simulink model "psc"  (R2023b)
settings: Solver=VariableStepAuto  StartTime=0.0  StopTime=.1  RelTol=1e-3
undefined symbols (not defined in the file): DiscIntNeverNeededParam, f_sw, K_p, L_f, L_g, R_a, R_L, T_s, U_dc, u_gN, w_b, w_g
libraries: simulink x1
settings Model: Creator=maatt  LastModifiedBy=maatt
settings DataIOCC: ReturnWorkspaceOutputs=off

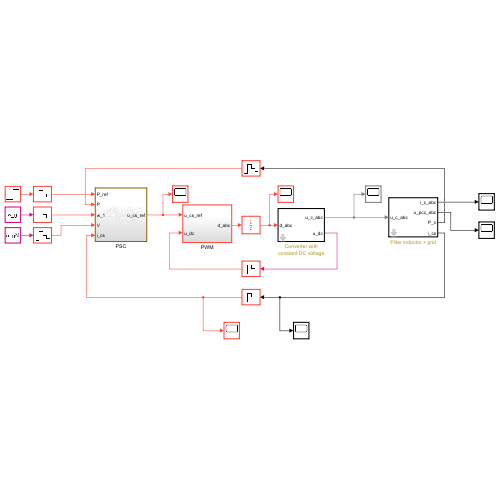
[thumbnail: Simulink's stored preview of the top-level diagram]
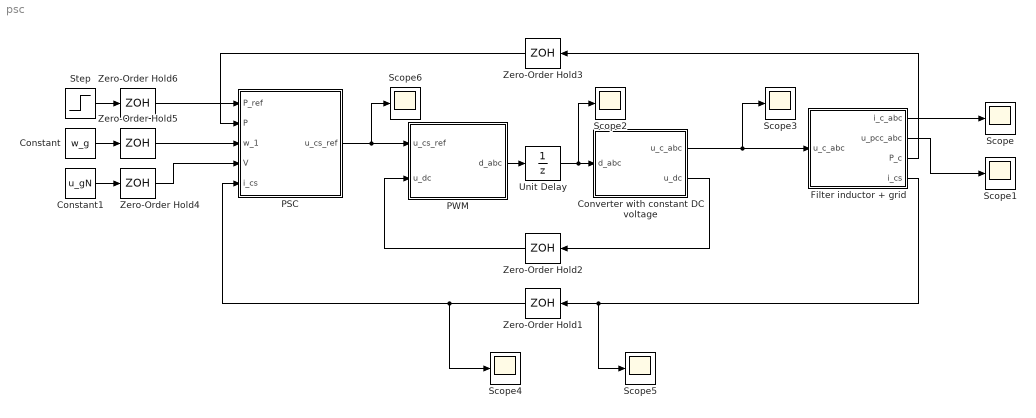
== system psc ==
  Constant : Constant  Value=w_g
  Constant1 : Constant  Value=u_gN
  "Converter with constant DC voltage " : Subsystem  mask{f_sw=f_sw, u_dc=U_dc}
      mask prompts: f_sw "Switching frequency (Hz)"; u_dc "DC-bus voltage (V)"
      mask init:
      | T_s = 1/(2*f_sw);
  Filter inductor + grid : Subsystem  mask{L_f=L_f, L_g=L_g, R_L=R_L}
      mask prompts: L_f "Filter inductance (H)"; L_g "Grid inductance (H)"; R_L "Series resistance (ohm)"
  PSC : Subsystem
  PWM : Subsystem
  Scope{,1..6} (7 alike) : Scope
  Step : Step  Time=.04  After=20  SampleTime=T_s
  Unit Delay : UnitDelay  SampleTime=T_s  HasFrameUpgradeWarning=on
  Zero-Order Hold{1..6} (6 alike) : ZeroOrderHold  SampleTime=T_s
  wires:
  "Converter with constant DC voltage "/1(u_c_abc) -> Scope3/1, Filter inductor + grid/1(u_c_abc)
  PWM/1(d_abc) -> Unit Delay/1
  PSC/1(u_cs_ref) -> Scope6/1, PWM/1(u_cs_ref)
  "Converter with constant DC voltage "/2(u_dc) -> Zero-Order Hold2/1
  Step/1 -> Zero-Order Hold6/1
  Constant/1 -> Zero-Order Hold5/1
  Constant1/1 -> Zero-Order Hold4/1
  Filter inductor + grid/1(i_c_abc) -> Scope/1
  Filter inductor + grid/2(u_pcc_abc) -> Scope1/1
  Filter inductor + grid/3(P_c) -> Zero-Order Hold3/1
  Filter inductor + grid/4(i_cs) -> Scope5/1, Zero-Order Hold1/1
  Unit Delay/1 -> Scope2/1, "Converter with constant DC voltage "/1(d_abc)
  Zero-Order Hold1/1 -> Scope4/1, PSC/5(i_cs)
  Zero-Order Hold2/1 -> PWM/2(u_dc)
  Zero-Order Hold3/1 -> PSC/2(P)
  Zero-Order Hold4/1 -> PSC/4(V)
  Zero-Order Hold5/1 -> PSC/3(w_1)
  Zero-Order Hold6/1 -> PSC/1(P_ref)

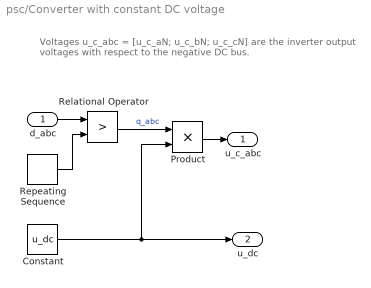
== system psc/Converter with constant DC voltage  ==
  note: Voltages u_c_abc = [u_c_aN; u_c_bN; u_c_cN] are the inverter
      | output voltages with respect to the negative DC bus.
  d_abc : Inport
  Constant : Constant  Value=u_dc
  Product : Product
  Relational Operator : RelationalOperator  Operator=>  OutDataTypeStr='double'  InputSameDT=off
  Repeating Sequence : simulink/Sources/Repeating Sequence  rep_seq_t=[0 1 2]*T_s  rep_seq_y=[1 0 1]
  u_c_abc : Outport
  u_dc : Outport  Port=2
  wires:
  Repeating Sequence/1 -> Relational Operator/2
  d_abc/1 -> Relational Operator/1
  Product/1 -> u_c_abc/1
  Relational Operator/1 -> Product/1  "q_abc"
  Constant/1 -> Product/2, u_dc/1

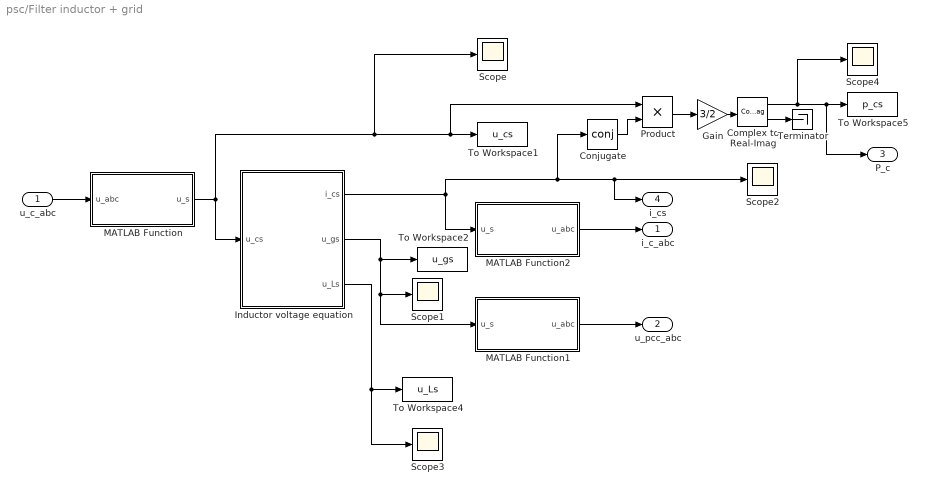
== system psc/Filter inductor + grid ==
  u_c_abc : Inport
  Complex to Real-Imag : ComplexToRealImag
  Conjugate : Math  Operator=conj  SignedPower=on  RndMeth=Zero
  Gain : Gain  Gain=3/2
  Inductor voltage equation : Subsystem
  MATLAB Function : MATLAB Function  TreatAsAtomicUnit=on
  MATLAB Function1 : MATLAB Function  TreatAsAtomicUnit=on
  MATLAB Function2 : MATLAB Function  TreatAsAtomicUnit=on
  Product : Product
  Scope{,1..4} (5 alike) : Scope
  Terminator : Terminator
  To Workspace1 : ToWorkspace  VariableName=u_cs  SaveFormat=Timeseries
  To Workspace2 : ToWorkspace  VariableName=u_gs  SaveFormat=Timeseries
  To Workspace4 : ToWorkspace  VariableName=u_Ls  SaveFormat=Timeseries
  To Workspace5 : ToWorkspace  VariableName=p_cs  SaveFormat=Timeseries
  i_c_abc : Outport
  u_pcc_abc : Outport  Port=2
  P_c : Outport  Port=3
  i_cs : Outport  Port=4
  wires:
  u_c_abc/1 -> MATLAB Function/1(u_abc)
  Inductor voltage equation/1(i_cs) -> i_cs/1, Scope2/1, Conjugate/1, MATLAB Function2/1(u_s)
  MATLAB Function2/1(u_abc) -> i_c_abc/1
  MATLAB Function/1(u_s) -> Inductor voltage equation/1(u_cs), Scope/1, Product/1, To Workspace1/1
  Inductor voltage equation/2(u_gs) -> Scope1/1, MATLAB Function1/1(u_s), To Workspace2/1
  Inductor voltage equation/3(u_Ls) -> To Workspace4/1, Scope3/1
  MATLAB Function1/1(u_abc) -> u_pcc_abc/1
  Conjugate/1 -> Product/2
  Complex to Real-Imag/1 -> Scope4/1, P_c/1, To Workspace5/1
  Complex to Real-Imag/2 -> Terminator/1
  Product/1 -> Gain/1
  Gain/1 -> Complex to Real-Imag/1

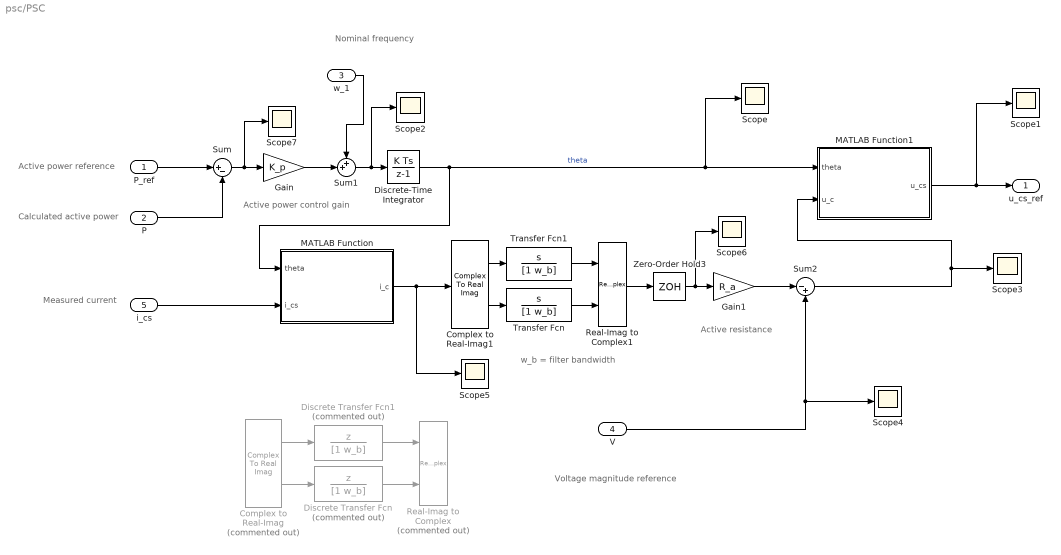
== system psc/PSC ==
  note: Active resistance
  note: Active power reference
  note: Calculated active power
  note: Measured current
  note: Nominal frequency
  note: Voltage magnitude reference
  note: Active power control gain
  note: w_b = filter bandwidth
  P_ref : Inport
  P : Inport  Port=2
  w_1 : Inport  Port=3
  V : Inport  Port=4
  i_cs : Inport  Port=5
  Complex to Real-Imag : ComplexToRealImag  Commented=on
  Complex to Real-Imag1 : ComplexToRealImag
  Discrete Transfer Fcn : DiscreteTransferFcn  Commented=on  Numerator=[1 0]  Denominator=[1 w_b]
  Discrete Transfer Fcn1 : DiscreteTransferFcn  Commented=on  Numerator=[1 0]  Denominator=[1 w_b]
  Discrete-Time Integrator : DiscreteIntegrator  SampleTime=T_s  OutMin=[-pi]  OutMax=[pi]  ICPrevOutput=DiscIntNeverNeededParam  ICPrevScaledInput=DiscIntNeverNeededParam
  Gain : Gain  Gain=K_p
  Gain1 : Gain  Gain=R_a
  MATLAB Function : MATLAB Function  TreatAsAtomicUnit=on
  MATLAB Function1 : MATLAB Function  TreatAsAtomicUnit=on
  Real-Imag to Complex : RealImagToComplex  Commented=on
  Real-Imag to Complex1 : RealImagToComplex
  Scope{,1..7} (8 alike) : Scope
  Sum : Sum  Inputs=|+-
  Sum1 : Sum  Inputs=++|
  Sum2 : Sum  Inputs=|-+
  Transfer Fcn : TransferFcn  Numerator=[1 0]  Denominator=[1 w_b]
  Transfer Fcn1 : TransferFcn  Numerator=[1 0]  Denominator=[1 w_b]
  Zero-Order Hold3 : ZeroOrderHold  SampleTime=T_s
  u_cs_ref : Outport
  wires:
  P_ref/1 -> Sum/1
  P/1 -> Sum/2
  Sum/1 -> Scope7/1, Gain/1
  Gain/1 -> Sum1/2
  w_1/1 -> Sum1/1
  Sum1/1 -> Discrete-Time Integrator/1, Scope2/1
  Discrete-Time Integrator/1 -> Scope/1, MATLAB Function1/1(theta), MATLAB Function/1(theta)  "theta"
  Gain1/1 -> Sum2/1
  V/1 -> Scope4/1, Sum2/2
  Sum2/1 -> MATLAB Function1/2(u_c), Scope3/1
  MATLAB Function1/1(u_cs) -> Scope1/1, u_cs_ref/1
  i_cs/1 -> MATLAB Function/2(i_cs)
  Complex to Real-Imag/1 -> Discrete Transfer Fcn1/1
  Complex to Real-Imag/2 -> Discrete Transfer Fcn/1
  MATLAB Function/1(i_c) -> Complex to Real-Imag1/1, Scope5/1
  Discrete Transfer Fcn/1 -> Real-Imag to Complex/2
  Discrete Transfer Fcn1/1 -> Real-Imag to Complex/1
  Transfer Fcn1/1 -> Real-Imag to Complex1/1
  Transfer Fcn/1 -> Real-Imag to Complex1/2
  Complex to Real-Imag1/2 -> Transfer Fcn/1
  Complex to Real-Imag1/1 -> Transfer Fcn1/1
  Zero-Order Hold3/1 -> Scope6/1, Gain1/1
  Real-Imag to Complex1/1 -> Zero-Order Hold3/1

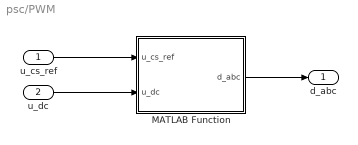
== system psc/PWM ==
  u_cs_ref : Inport
  u_dc : Inport  Port=2
  MATLAB Function : MATLAB Function  TreatAsAtomicUnit=on
  d_abc : Outport
  wires:
  u_cs_ref/1 -> MATLAB Function/1(u_cs_ref)
  MATLAB Function/1(d_abc) -> d_abc/1
  u_dc/1 -> MATLAB Function/2(u_dc)

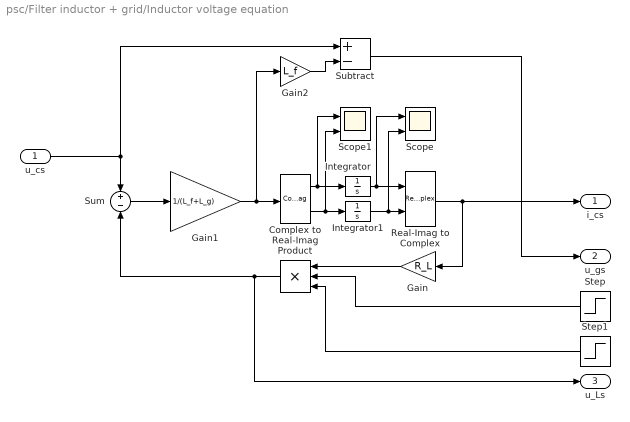
== system psc/Filter inductor + grid/Inductor voltage equation ==
  u_cs : Inport
  Complex to Real-Imag : ComplexToRealImag
  Gain : Gain  Gain=R_L
  Gain1 : Gain  Gain=1/(L_f+L_g)
  Gain2 : Gain  Gain=L_f
  Integrator : Integrator
  Integrator1 : Integrator
  Product : Product  Inputs=3
  Real-Imag to Complex : RealImagToComplex
  Scope : Scope  NumInputPorts=2
  Scope1 : Scope  NumInputPorts=2
  Step : Step  Time=0.05  Before=1  After=2  SampleTime=0
  Step1 : Step  Time=0.08  Before=1  SampleTime=0
  Subtract : Sum  Inputs=+-
  Sum : Sum  Inputs=+|-
  i_cs : Outport
  u_gs : Outport  Port=2
  u_Ls : Outport  Port=3
  wires:
  u_cs/1 -> Subtract/1, Sum/1
  Sum/1 -> Gain1/1
  Gain1/1 -> Gain2/1, Complex to Real-Imag/1
  Complex to Real-Imag/1 -> Scope1/1, Integrator/1
  Complex to Real-Imag/2 -> Scope1/2, Integrator1/1
  Integrator/1 -> Scope/1, Real-Imag to Complex/1
  Integrator1/1 -> Scope/2, Real-Imag to Complex/2
  Real-Imag to Complex/1 -> i_cs/1, Gain/1
  Gain/1 -> Product/1
  Gain2/1 -> Subtract/2
  Subtract/1 -> u_gs/1
  Step/1 -> Product/2
  Product/1 -> u_Ls/1, Sum/2
  Step1/1 -> Product/3

== matlab function psc/PSC/MATLAB Function1 ==
  data: theta input size=1; u_c input size=1; u_cs output size=1
function u_cs = dq2alphabeta(theta, u_c)

% % Space-vector transformation
% i_cs = 2/3*(i_c_abc(1) + i_c_abc(2)*exp(1j*2*pi/3) ...
%     + i_c_abc(3)*exp(1j*4*pi/3));

% Coordinate transformation
u_cs = u_c*exp(1j*theta);

== matlab function psc/PWM/MATLAB Function ==
  data: d_abc output; u_cs_ref input; u_dc input
function d_abc = fcn(u_cs_ref, u_dc)

%% Symmetrical suboscillation PWM
% Components of the voltage space vector
u_c_alpha_ref = real(u_cs_ref);
u_c_beta_ref  = imag(u_cs_ref);

% Phase-voltage references
u_ca_ref = u_c_alpha_ref;
u_cb_ref = .5*(-u_c_alpha_ref + sqrt(3)*u_c_beta_ref);
u_cc_ref = .5*(-u_c_alpha_ref - sqrt(3)*u_c_beta_ref);

% Vector of phase-voltage references
u_c_abc_ref = [u_ca_ref; u_cb_ref; u_cc_ref];

% Symmetrization of the references by adding the zero-sequence voltage
u0 = .5*(max(u_c_abc_ref) + min(u_c_abc_ref));
u_c_abc_ref = u_c_abc_ref - u0;

% Clipping of the reference voltages such that no phase error is caused. 
% If all phase voltage reference are realizable (below u_dc/2), m = 1 holds.
m = max([2*u_c_abc_ref/u_dc; 1]);
u_c_abc_ref = u_c_abc_ref/m;

% Duty cycles, which can be directly used for triangle comparison, 
% if the triangle wave varies between 0...1
d_abc = .5 + u_c_abc_ref/u_dc;
% 
% % Realized voltage vector is calculated from the clamped duty ratios.
% % If the PWM does not saturate, u_c_ref_lim = u_c_ref holds. The realized
% % voltage vector is needed, e.g., for the current-controller antiwindup.
% u_cs_ref_lim = 2/3*(d_abc(1) + d_abc(2)*exp(1j*2*pi/3) ...
%     + d_abc(3)*exp(1j*4*pi/3))*u_dc;
% % In estimated rotor flux coordinates
% u_c_ref_lim = exp(-1j*theta)*u_cs_ref_lim;

== matlab function psc/Filter inductor + grid/MATLAB Function1 ==
  data: u_s input size=1; u_abc output size=3
function u_abc = s2abc(u_s)

% Inverse space-vector transformation
u_abc = real([1; exp(-1j*2*pi/3); exp(-1j*4*pi/3)]*u_s);

== matlab function psc/PSC/MATLAB Function ==
  data: theta input size=1; i_cs input; i_c output size=1
function i_c = alphabeta2dq(theta, i_cs)

% % Space-vector transformation
% i_cs = 2/3*(i_c_abc(1) + i_c_abc(2)*exp(1j*2*pi/3) ...
%     + i_c_abc(3)*exp(1j*4*pi/3));

% Coordinate transformation
i_c = i_cs*exp(-1j*theta);

== matlab function psc/Filter inductor + grid/MATLAB Function ==
  data: u_abc input size=3; u_s output size=1
function u_s = abc2s(u_abc)

% Space-vector transformation
u_s = 2/3*(u_abc(1) + u_abc(2)*exp(1j*2*pi/3) + u_abc(3)*exp(1j*4*pi/3));

== matlab function psc/Filter inductor + grid/MATLAB Function2 ==
  data: u_s input size=1; u_abc output size=3
function u_abc = s2abc(u_s)

% Inverse space-vector transformation
u_abc = real([1; exp(-1j*2*pi/3); exp(-1j*4*pi/3)]*u_s);
